simulink model "FP_PMSM_ProposedDTC"  (R2023b)
settings: Solver=ode1  StartTime=0.0  StopTime=2  FixedStep=140e-6  RelTol=1e-3
undefined symbols (not defined in the file): J, Lamda_PM, Lls, Ls, Mod_Lamda_s_ref, P, Rs
libraries: spsPWMGeneratorDCDCLib x1, spspowerguiLib x1
(part 1 of 2)
settings Model: SimulationMode=rapid-accelerator  Creator=rajan  LastModifiedBy=rajan
settings SolverCC: AlgebraicLoopSolver=TrustRegion
settings DataIOCC: ReturnWorkspaceOutputs=off
settings OptimizationCC: BlockReduction=off
settings DebuggingCC: AlgebraicLoopMsg=none  UnconnectedInputMsg=warning  UnconnectedOutputMsg=warning  UnconnectedLineMsg=warning  ArithmeticOperatorsInVariantConditions=warning
settings ModelReferenceCC: EnableRefExpFcnMdlSchedulingChecks=on
settings SFSimCC: SimUseLocalCustomCode=off  CustomCodeUndefinedFunction=UseInterfaceOnly
settings RTWCC: RTWUseLocalCustomCode=off
settings CodeAppCC: StateflowObjectComments=on
settings SimscapeCC: SimscapeNormalizeSystem=off

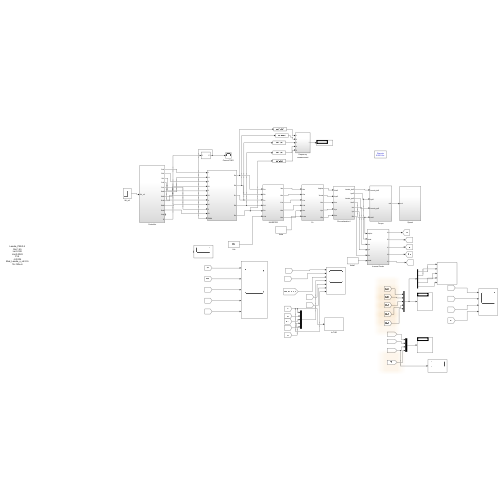
[thumbnail: Simulink's stored preview of the top-level diagram]
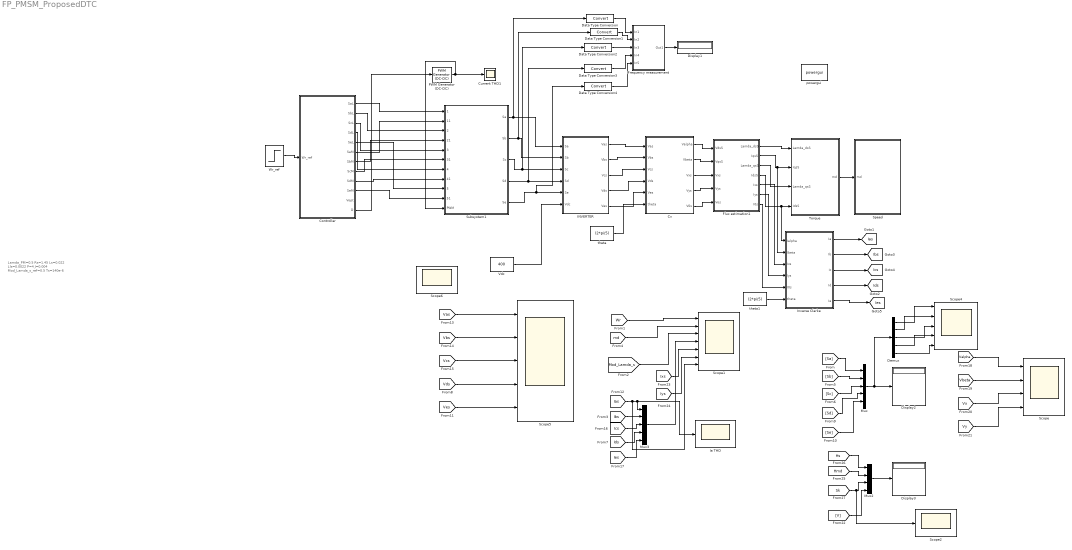
== system FP_PMSM_ProposedDTC ==
  note: Lamda_PM=0.5
      | Rs=1.45
      | Ls=0.022
      | Lls=0.0022
      | P=4
      | J=0.004
      | Mod_Lamda_s_ref=0.5
      | Ts=140e-6
  Controller : Subsystem
  Current THD1 : Scope
  "Cv " : Subsystem
  Data Type Conversion{,1..4} (5 alike) : DataTypeConversion  SaturateOnIntegerOverflow=off  RndMeth=Floor
  Demux : Demux  Outputs=5
  Display1 : Display
  Display2 : Display
  Display3 : Display
  Flux estimation1 : Subsystem
  Frequency measurement : Subsystem
  INVERTER : Subsystem
  Ia THD : Scope
  Inverse Clarke : Subsystem
  Mux : Mux  Inputs=5
  Mux2 : Mux
  Mux3 : Mux  Inputs=5
  PWM Generator (DC-DC) : spsPWMGeneratorDCDCLib/PWM Generator (DC-DC)  Fsw=3000  Ts=140e-6
  Scope : Scope  NumInputPorts=4
  Scope1 : Scope  NumInputPorts=7
  Scope2 : Scope
  Scope4 : Scope  NumInputPorts=5
  Scope5 : Scope  NumInputPorts=5
  Scope6 : Scope
  Speed : Subsystem
  Subsystem1 : Subsystem
  Torque : Subsystem
  Vdc : Constant  Value=400
  Wr_ref : Step  Time=0.5  Before=104.7197  After=104.7197  SampleTime=0  VectorParams1D=off
  powergui : spspowerguiLib/powergui  Priority=1  SimulationMode=Discrete  SampleTime=140e-6  frequency=60  Iterations=50  frequencyindice=60  Pbase=100e6  ErrMax=1e-4  UnitsV=kV  UnitsW=MW  buscounter=0  FunctionMessages=off  echomessages=off  EnableUseOfTLC=off  CurrentSourceSwitches=off  DisableSnubberDevices=off  DisableRonSwitches=off  DisableVfSwitches=off  DisplayEquations=off  AutomaticDiscreteSolvers=off  SolverType=Tustin/Backward Euler (TBE)  Interpol=off  ExternalGateDelay=off  methode=off  Ts=10  x0status=blocks  SPID=off  SwTol=0  HookPort=off  NonlinearTolerance=1e-4  nMaxIteration=100  ContinueOnMaxIteration=off  RestoreLinks=warning  ResistiveCurrentMeasurement=off  Frange=[0:2:500]  Ylog=off  Xlog=on  ShowGrid=off  save=off  variable=ZData  structure=Ia_THD  ZoomFFT=off  StartTime=0.15  cycles=10  DisplayStyle=2  fundamental=31.83  FreqAxis=off  MaxFrequency=1000  frequencyindicesteady=1  RmsSteady=1  display=off
  theta : Constant  Value=(2*pi/5)
  theta1 : Constant  Value=(2*pi/5)
  tag scope: Ias=global, Ibs=global, Ics=global, Ids=global, Ies=global
  wires:
  [Vbs] -> Scope5/2
  [Vas] -> Scope5/1
  [Vcs] -> Scope5/3
  [Wr] -> Scope1/1
  [md] -> Scope1/2
  [Mod_Lamda_s] -> Scope1/3
  Mux2/1 -> Display3/1
  [V] -> Mux2/4
  [Hmd] -> Mux2/2
  [Hs] -> Mux2/1
  [Sk] -> Scope2/1, Mux2/3
  [Ics] -> Mux3/3
  [Ias] -> Scope1/7, Mux3/1, Ia THD/1
  [Ibs] -> Mux3/2
  [Ids] -> Mux3/4
  [Ies] -> Mux3/5
  Mux3/1 -> Scope1/4
  INVERTER/1(Vas) -> "Cv "/1(Vas)
  INVERTER/2(Vbs) -> "Cv "/2(Vbs)
  INVERTER/3(Vcs) -> "Cv "/3(Vcs)
  INVERTER/4(Vds) -> "Cv "/4(Vds)
  INVERTER/5(Ves) -> "Cv "/5(Ves)
  "Cv "/1(Valpha) -> Flux estimation1/1(VdsS)
  "Cv "/2(Vbeta) -> Flux estimation1/2(VqsS)
  Flux estimation1/1(Lamda_dsS) -> Torque/1(Lamda_dsS)
  Flux estimation1/2(IqsS) -> Torque/2(IqsS), Inverse Clarke/2(Ibeta)
  Flux estimation1/3(Lamda_qsS) -> Torque/3(Lamda_qsS)
  Flux estimation1/4(IdsS) -> Inverse Clarke/1(Ialpha), Torque/4(IdsS)
  Torque/1(md) -> Speed/1(md)
  Wr_ref/1 -> Controller/1(Wr_ref)
  [Vds] -> Scope5/4
  [Ves] -> Scope5/5
  Vdc/1 -> INVERTER/6(Vdc)
  theta/1 -> "Cv "/6(theta)
  "Cv "/3(Vxs) -> Flux estimation1/3(Vxs)
  "Cv "/4(Vys) -> Flux estimation1/4(Vys)
  "Cv "/5(V0s) -> Flux estimation1/5(Vos)
  [Valpha] -> Scope/1
  [Vbeta] -> Scope/2
  [Vx] -> Scope/3
  [Vy] -> Scope/4
  [Ixs] -> Scope1/5
  [Iys] -> Scope1/6
  Flux estimation1/5(Ixs) -> Inverse Clarke/3(Ixs)
  Flux estimation1/6(Iys) -> Inverse Clarke/4(Iys)
  Flux estimation1/7(I0s) -> Inverse Clarke/5(I0s)
  theta1/1 -> Inverse Clarke/6(theta)
  Inverse Clarke/1(Ia) -> [Ias]
  Inverse Clarke/2(Ib) -> [Ibs]
  Inverse Clarke/3(Ic) -> [Ics]
  Inverse Clarke/4(Id) -> [Ids]
  Inverse Clarke/5(Ie) -> [Ies]
  [Sa] -> Mux/1
  [Sb] -> Mux/2
  [Sc] -> Mux/3
  Mux/1 -> Demux/1, Display2/1
  [Sd] -> Mux/4
  [Se] -> Mux/5
  Demux/1 -> Scope4/1
  Demux/2 -> Scope4/2
  Demux/3 -> Scope4/3
  Demux/4 -> Scope4/4
  Demux/5 -> Scope4/5
  PWM Generator (DC-DC)/1 -> Subsystem1/11(PWM), Current THD1/1
  Controller/1(SaL) -> Subsystem1/1(1)
  Controller/2(SbL) -> Subsystem1/3(2)
  Controller/3(ScL) -> Subsystem1/5(3)
  Controller/4(SdL) -> Subsystem1/7(4)
  Controller/5(SeL) -> Subsystem1/9(5)
  Controller/6(SaM) -> Subsystem1/2(11)
  Controller/7(SbM) -> Subsystem1/4(21)
  Controller/8(ScM) -> Subsystem1/6(31)
  Controller/9(SdM) -> Subsystem1/8(41)
  Controller/10(SeM) -> Subsystem1/10(51)
  Controller/12(D) -> PWM Generator (DC-DC)/1
  Subsystem1/1(Sa) -> Data Type Conversion/1, INVERTER/1(Sa)
  Subsystem1/2(Sb) -> Data Type Conversion1/1, INVERTER/2(Sb)
  Subsystem1/3(Sc) -> Data Type Conversion2/1, INVERTER/3(Sc)
  Subsystem1/4(Sd) -> Data Type Conversion3/1, INVERTER/4(Sd)
  Subsystem1/5(Se) -> Data Type Conversion4/1, INVERTER/5(Se)
  Frequency measurement/1(Out1) -> Display1/1
  Data Type Conversion/1 -> Frequency measurement/1(In1)
  Data Type Conversion1/1 -> Frequency measurement/2(In2)
  Data Type Conversion2/1 -> Frequency measurement/3(In3)
  Data Type Conversion3/1 -> Frequency measurement/4(In4)
  Data Type Conversion4/1 -> Frequency measurement/5(In5)

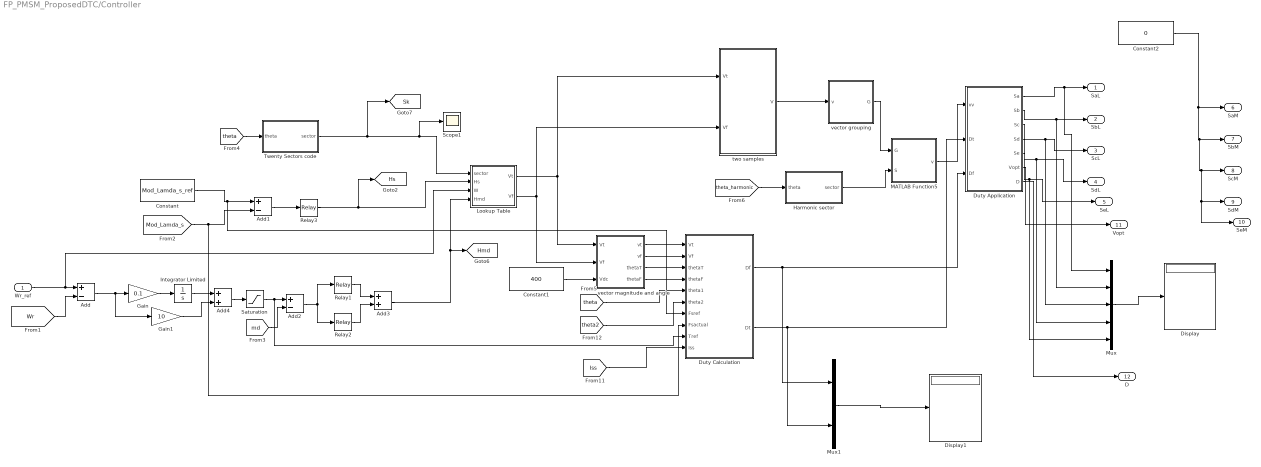
== system FP_PMSM_ProposedDTC/Controller ==
  Wr_ref : Inport
  Add : Sum  Inputs=+-
  Add1 : Sum  Inputs=+-
  Add2 : Sum  Inputs=+-
  Add3 : Sum
  Add4 : Sum
  Constant : Constant  Value=Mod_Lamda_s_ref
  Constant1 : Constant  Value=400
  Constant2 : Constant  Value=0
  Display : Display
  Display1 : Display
  Duty Application : MATLAB Function  TreatAsAtomicUnit=on
  Duty Calculation : MATLAB Function  TreatAsAtomicUnit=on
  Gain : Gain  Gain=0.1
  Gain1 : Gain  Gain=10
  "Harmonic sector " : MATLAB Function  TreatAsAtomicUnit=on
  Integrator Limited : Integrator  LimitOutput=on  UpperSaturationLimit=14  LowerSaturationLimit=-14
  Lookup Table : MATLAB Function  TreatAsAtomicUnit=on
  MATLAB Function5 : MATLAB Function  TreatAsAtomicUnit=on
  Mux : Mux  Inputs=5
  Mux1 : Mux  Inputs=2
  Relay1 : Relay  OnSwitchValue=1.4  OffSwitchValue=0
  Relay2 : Relay  OnSwitchValue=0  OffSwitchValue=-1.4  OnOutputValue=0  OffOutputValue=-1
  Relay3 : Relay  OnSwitchValue=0.005  OffSwitchValue=-0.005  OffOutputValue=-1
  Saturation : Saturate  UpperLimit=14  LowerLimit=-14
  Scope1 : Scope
  Twenty Sectors code : MATLAB Function  TreatAsAtomicUnit=on
  two samples : MATLAB Function  TreatAsAtomicUnit=on
  vector grouping : MATLAB Function  TreatAsAtomicUnit=on
  vector magnitude and angle : Subsystem
  SaL : Outport
  SbL : Outport  Port=2
  ScL : Outport  Port=3
  SdL : Outport  Port=4
  SeL : Outport  Port=5
  SaM : Outport  Port=6
  SbM : Outport  Port=7
  ScM : Outport  Port=8
  SdM : Outport  Port=9
  SeM : Outport  Port=10
  Vopt : Outport  Port=11
  D : Outport  Port=12
  tag scope: Hmd=global, Hs=global, Sk=global
  wires:
  Gain1/1 -> Add4/2
  Integrator Limited/1 -> Add4/1
  [md] -> Add2/2
  Gain/1 -> Integrator Limited/1
  Relay2/1 -> Add3/2
  [Wr] -> Add/2
  Add1/1 -> Relay3/1
  Relay3/1 -> Lookup Table/2(Hs), [Hs]
  [theta] -> Twenty Sectors code/1(theta)
  Constant/1 -> Duty Calculation/7(Fsref), Add1/1
  Add3/1 -> Lookup Table/4(Hmd), [Hmd]
  [Mod_Lamda_s] -> Duty Calculation/8(Fsactual), Add1/2
  Add2/1 -> Relay1/1, Relay2/1
  Relay1/1 -> Add3/1
  Add/1 -> Gain1/1, Gain/1
  Saturation/1 -> Duty Calculation/9(Tref), Add2/1
  Add4/1 -> Saturation/1
  Wr_ref/1 -> Lookup Table/3(W), Add/1
  Twenty Sectors code/1(sector) -> [Sk], Lookup Table/1(sector), Scope1/1
  Lookup Table/1(Vt) -> vector magnitude and angle/1(Vt), two samples/1(Vt)
  Lookup Table/2(Vf) -> vector magnitude and angle/2(Vf), two samples/2(Vf)
  Constant1/1 -> vector magnitude and angle/3(Vdc)
  vector magnitude and angle/1(vt) -> Duty Calculation/1(Vt)
  vector magnitude and angle/2(vf) -> Duty Calculation/2(Vf)
  vector magnitude and angle/3(thetaT) -> Duty Calculation/3(thetaT)
  vector magnitude and angle/4(thetaF) -> Duty Calculation/4(thetaF)
  [theta] -> Duty Calculation/5(theta1)
  [theta2] -> Duty Calculation/6(theta2)
  [Iss] -> Duty Calculation/10(Iss)
  "Harmonic sector "/1(sector) -> MATLAB Function5/2(S)
  vector grouping/1(G) -> MATLAB Function5/1(G)
  MATLAB Function5/1(v) -> Duty Application/1(vv)
  [theta_harmonic] -> "Harmonic sector "/1(theta)
  two samples/1(V) -> vector grouping/1(v)
  Duty Application/1(Sa) -> Mux/1, SaL/1
  Duty Application/2(Sb) -> Mux/2, SbL/1
  Duty Application/3(Sc) -> Mux/3, ScL/1
  Duty Application/4(Sd) -> Mux/4, SdL/1
  Duty Application/5(Se) -> Mux/5, SeL/1
  Duty Calculation/2(Dt) -> Mux1/2, Duty Application/2(Dt)
  Duty Calculation/1(Df) -> Mux1/1, Duty Application/3(Df)
  Mux/1 -> Display/1
  Mux1/1 -> Display1/1
  Duty Application/6(Vopt) -> Vopt/1
  Constant2/1 -> SeM/1, SdM/1, ScM/1, SbM/1, SaM/1
  Duty Application/7(D) -> D/1

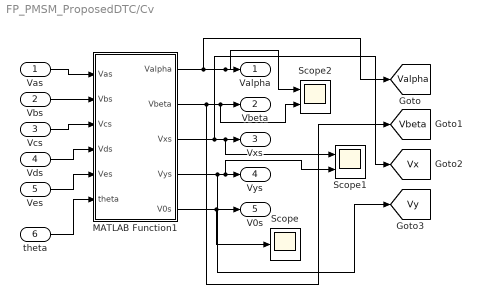
== system FP_PMSM_ProposedDTC/Cv  ==
  Vas : Inport
  Vbs : Inport  Port=2
  Vcs : Inport  Port=3
  Vds : Inport  Port=4
  Ves : Inport  Port=5
  theta : Inport  Port=6
  MATLAB Function1 : MATLAB Function  TreatAsAtomicUnit=on
  Scope : Scope
  Scope1 : Scope  NumInputPorts=2
  Scope2 : Scope  NumInputPorts=2
  Valpha : Outport
  Vbeta : Outport  Port=2
  Vxs : Outport  Port=3
  Vys : Outport  Port=4
  V0s : Outport  Port=5
  tag scope: Valpha=global, Vbeta=global, Vx=global, Vy=global
  wires:
  Vas/1 -> MATLAB Function1/1(Vas)
  Vbs/1 -> MATLAB Function1/2(Vbs)
  Ves/1 -> MATLAB Function1/5(Ves)
  Vcs/1 -> MATLAB Function1/3(Vcs)
  Vds/1 -> MATLAB Function1/4(Vds)
  theta/1 -> MATLAB Function1/6(theta)
  MATLAB Function1/1(Valpha) -> [Valpha], Scope2/1, Valpha/1
  MATLAB Function1/2(Vbeta) -> [Vbeta], Scope2/2, Vbeta/1
  MATLAB Function1/3(Vxs) -> [Vx], Scope1/1, Vxs/1
  MATLAB Function1/4(Vys) -> Vys/1, Scope1/2, [Vy]
  MATLAB Function1/5(V0s) -> Scope/1, V0s/1

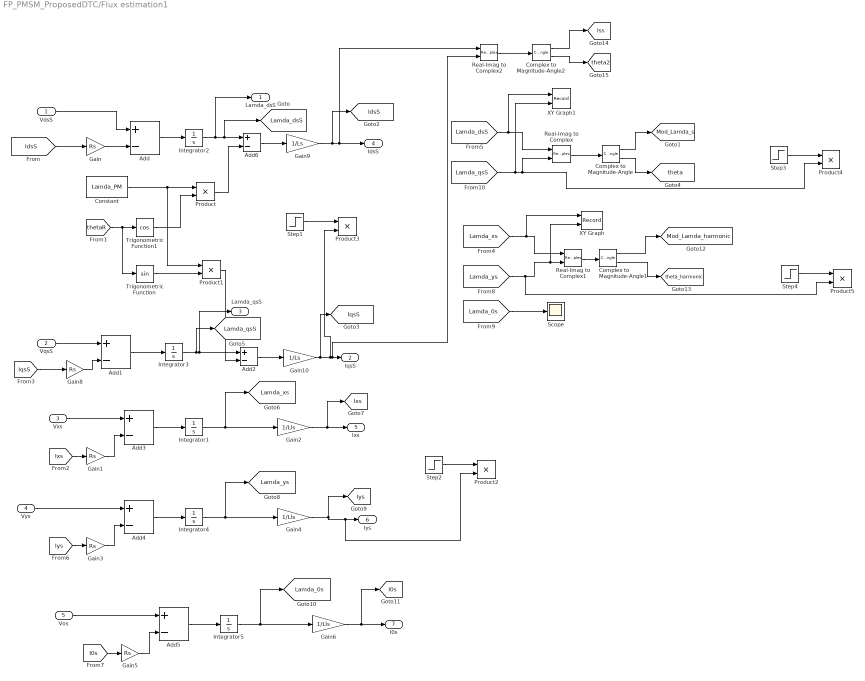
== system FP_PMSM_ProposedDTC/Flux estimation1 ==
  VdsS : Inport
  VqsS : Inport  Port=2
  Vxs : Inport  Port=3
  Vys : Inport  Port=4
  Vos : Inport  Port=5
  Add{,1..6} (7 alike) : Sum  Inputs=+-
  Complex to Magnitude-Angle : ComplexToMagnitudeAngle
  Complex to Magnitude-Angle1 : ComplexToMagnitudeAngle
  Complex to Magnitude-Angle2 : ComplexToMagnitudeAngle
  Constant : Constant  Value=Lamda_PM
  Gain{,1,3,5,8} (5 alike) : Gain  Gain=Rs
  Gain10 : Gain  Gain=1/Ls
  Gain2 : Gain  Gain=1/Lls
  Gain4 : Gain  Gain=1/Lls
  Gain6 : Gain  Gain=1/Lls
  Gain9 : Gain  Gain=1/Ls
  Integrator{1..5} (5 alike) : Integrator  UpperSaturationLimit=0.5  LowerSaturationLimit=-0.5
  Product{,1..5} (6 alike) : Product
  Real-Imag to Complex : RealImagToComplex
  Real-Imag to Complex1 : RealImagToComplex
  Real-Imag to Complex2 : RealImagToComplex
  Scope : Scope
  Step{1..4} (4 alike) : Step  Time=0.5  SampleTime=0
  Trigonometric Function : Trigonometry
  Trigonometric Function1 : Trigonometry  Operator=cos
  XY Graph : Record  FileSettingsInternal="{\"entries\":[{\"content\":{\"excelSettings\":{\"content\":{},\"type\":\"Streamout.ExcelSettings\"}},\"type\":\"Streamout.FileSettingStorage\",\"uuid\":\"\"}],\"packageUris\":[\"http:\\/\\/schema.mathworks.com\\/mf0\\/streamout_blocks\\/R2020a\"],\"version\":\"1.0\"}"  Layout=[1 1]  SignalsInternal="{\"entries\":[{\"content\":{\"signals\":[{\"content\":{\"blockPath\":[],\"dimensions\":[1],\"domain\":\"\",\"lineColor\":\"#a2142f\",\"plots\":[1],\"port\":1,\"signalID\":24,\"signalName\":\"XY Graph:1\"},\"type\":\"RecordBlkView.Signal\",\"uuid\":\"\"},{\"content\":{\"blockPath\":[],\"dimensions\":[1],\"domain\":\"\",\"lineColor\":\"#139fff\",\"plots\":[1],\"port\":2,\"signalID\":27,\"signalName\":\"XY Graph:2\"},\"type\":\"RecordBlkView.Signal\",\"uuid\":\"\"}]},\"type\":\"RecordBlkView.InputSignals\",\"uuid\":\"\"}],\"packageUris\":[\"http:\\/\\/schema.mathworks.com\\/mf0\\/streamout_blocks\\/R2020a\"],\"version\":\"1.0\"}"  VisualizationBindings="{\"xyplotplugin\":{\"info\":[{\"series\":[{\"bindingParametersList\":[{\"parameter\":\"X-Axis\",\"signalID\":24,\"signalName\":\"XY Graph:1\"},{\"parameter\":\"Y-Axis\",\"signalID\":27,\"signalName\":\"XY Graph:2\"}],\"seriesID\":36795}],\"subplotID\":1}]}}"  CompatibilityTag=XY  st=-1
  XY Graph1 : Record  FileSettingsInternal="{\"entries\":[{\"content\":{\"excelSettings\":{\"content\":{},\"type\":\"Streamout.ExcelSettings\"}},\"type\":\"Streamout.FileSettingStorage\",\"uuid\":\"\"}],\"packageUris\":[\"http:\\/\\/schema.mathworks.com\\/mf0\\/streamout_blocks\\/R2020a\"],\"version\":\"1.0\"}"  Layout=[1 1]  SignalsInternal="{\"entries\":[{\"content\":{\"signals\":[{\"content\":{\"blockPath\":[],\"dimensions\":[1],\"domain\":\"\",\"lineColor\":\"#a2142f\",\"plots\":[1],\"port\":1,\"signalID\":16,\"signalName\":\"XY Graph:1\"},\"type\":\"RecordBlkView.Signal\",\"uuid\":\"\"},{\"content\":{\"blockPath\":[],\"dimensions\":[1],\"domain\":\"\",\"lineColor\":\"#139fff\",\"plots\":[1],\"port\":2,\"signalID\":19,\"signalName\":\"XY Graph:2\"},\"type\":\"RecordBlkView.Signal\",\"uuid\":\"\"}]},\"type\":\"RecordBlkView.InputSignals\",\"uuid\":\"\"}],\"packageUris\":[\"http:\\/\\/schema.mathworks.com\\/mf0\\/streamout_blocks\\/R2020a\"],\"version\":\"1.0\"}"  VisualizationBindings="{\"xyplotplugin\":{\"info\":[{\"series\":[{\"bindingParametersList\":[{\"parameter\":\"X-Axis\",\"signalID\":16,\"signalName\":\"XY Graph:1\"},{\"parameter\":\"Y-Axis\",\"signalID\":19,\"signalName\":\"XY Graph:2\"}],\"seriesID\":10148}],\"subplotID\":1}]}}"  CompatibilityTag=XY  st=-1
  Lamda_dsS : Outport
  IqsS : Outport  Port=2
  Lamda_qsS : Outport  Port=3
  IdsS : Outport  Port=4
  Ixs : Outport  Port=5
  Iys : Outport  Port=6
  I0s : Outport  Port=7
  tag scope: I0s=global, IdsS=global, IqsS=global, Iss=global, Ixs=global, Iys=global, Lamda_0s=global, Lamda_dsS=global, Lamda_qsS=global, Lamda_xs=global, Lamda_ys=global, Mod_Lamda_harmonic=global, Mod_Lamda_s=global, theta2=global, theta=global, theta_harmonic=global
  wires:
  Real-Imag to Complex/1 -> Complex to Magnitude-Angle/1
  Complex to Magnitude-Angle/1 -> [Mod_Lamda_s]
  Add/1 -> Integrator2/1
  Integrator2/1 -> Lamda_dsS/1, [Lamda_dsS], Add6/1
  VqsS/1 -> Add1/1
  Add1/1 -> Integrator3/1
  Integrator3/1 -> [Lamda_qsS], Add2/1, Lamda_qsS/1
  Gain8/1 -> Add1/2
  [IdsS] -> Gain/1
  Gain/1 -> Add/2
  VdsS/1 -> Add/1
  [IqsS] -> Gain8/1
  Add6/1 -> Gain9/1
  Complex to Magnitude-Angle/2 -> [theta]
  Add2/1 -> Gain10/1
  [thetaR] -> Trigonometric Function/1, Trigonometric Function1/1
  Constant/1 -> Product1/1, Product/1
  Trigonometric Function1/1 -> Product/2
  Product/1 -> Add6/2
  Trigonometric Function/1 -> Product1/2
  Product1/1 -> Add2/2
  [Ixs] -> Gain1/1
  Gain1/1 -> Add3/2
  Vxs/1 -> Add3/1
  Add3/1 -> Integrator1/1
  Integrator1/1 -> [Lamda_xs], Gain2/1
  Add4/1 -> Integrator4/1
  Vys/1 -> Add4/1
  [Iys] -> Gain3/1
  Gain3/1 -> Add4/2
  Integrator4/1 -> [Lamda_ys], Gain4/1
  Gain5/1 -> Add5/2
  Gain6/1 -> I0s/1, [I0s]
  Vos/1 -> Add5/1
  Integrator5/1 -> [Lamda_0s], Gain6/1
  Add5/1 -> Integrator5/1
  [I0s] -> Gain5/1
  Complex to Magnitude-Angle1/1 -> [Mod_Lamda_harmonic]
  Complex to Magnitude-Angle1/2 -> [theta_harmonic]
  Real-Imag to Complex1/1 -> Complex to Magnitude-Angle1/1
  [Lamda_0s] -> Scope/1
  Step1/1 -> Product3/1
  Gain4/1 -> [Iys], Product2/2, Iys/1
  Step2/1 -> Product2/1
  Gain2/1 -> Ixs/1, [Ixs]
  [Lamda_qsS] -> XY Graph1/2, Product4/2, Real-Imag to Complex/2
  Step3/1 -> Product4/1
  [Lamda_dsS] -> XY Graph1/1, Real-Imag to Complex/1
  [Lamda_ys] -> Product5/2, XY Graph/2, Real-Imag to Complex1/2
  Step4/1 -> Product5/1
  [Lamda_xs] -> Real-Imag to Complex1/1, XY Graph/1
  Gain9/1 -> [IdsS], Real-Imag to Complex2/1, IdsS/1
  Gain10/1 -> [IqsS], Product3/2, Real-Imag to Complex2/2, IqsS/1
  Real-Imag to Complex2/1 -> Complex to Magnitude-Angle2/1
  Complex to Magnitude-Angle2/1 -> [Iss]
  Complex to Magnitude-Angle2/2 -> [theta2]

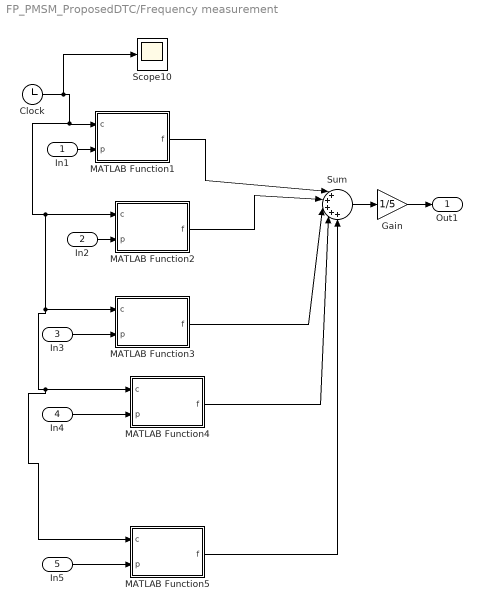
== system FP_PMSM_ProposedDTC/Frequency measurement ==
  In1 : Inport
  In2 : Inport  Port=2
  In3 : Inport  Port=3
  In4 : Inport  Port=4
  In5 : Inport  Port=5
  Clock : Clock
  Gain : Gain  Gain=1/5
  MATLAB Function1 : MATLAB Function  TreatAsAtomicUnit=on
  MATLAB Function2 : MATLAB Function  TreatAsAtomicUnit=on
  MATLAB Function3 : MATLAB Function  TreatAsAtomicUnit=on
  MATLAB Function4 : MATLAB Function  TreatAsAtomicUnit=on
  MATLAB Function5 : MATLAB Function  TreatAsAtomicUnit=on
  Scope10 : Scope
  Sum : Sum  Inputs=|+++++
  Out1 : Outport
  wires:
  MATLAB Function1/1(f) -> Sum/1
  In1/1 -> MATLAB Function1/2(p)
  MATLAB Function2/1(f) -> Sum/2
  In2/1 -> MATLAB Function2/2(p)
  MATLAB Function3/1(f) -> Sum/3
  In3/1 -> MATLAB Function3/2(p)
  Sum/1 -> Gain/1
  Gain/1 -> Out1/1
  MATLAB Function4/1(f) -> Sum/4
  In4/1 -> MATLAB Function4/2(p)
  Clock/1 -> Scope10/1, MATLAB Function5/1(c), MATLAB Function4/1(c), MATLAB Function3/1(c), MATLAB Function2/1(c), MATLAB Function1/1(c)
  MATLAB Function5/1(f) -> Sum/5
  In5/1 -> MATLAB Function5/2(p)

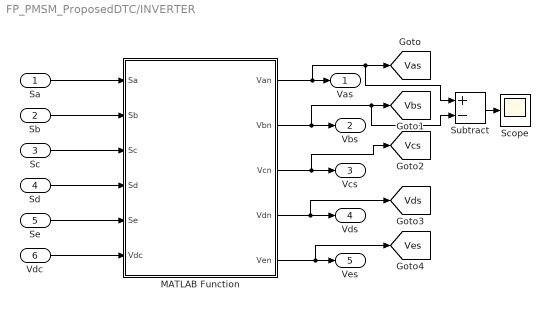
== system FP_PMSM_ProposedDTC/INVERTER ==
  Sa : Inport
  Sb : Inport  Port=2
  Sc : Inport  Port=3
  Sd : Inport  Port=4
  Se : Inport  Port=5
  Vdc : Inport  Port=6
  MATLAB Function : MATLAB Function  TreatAsAtomicUnit=on
  Scope : Scope
  Subtract : Sum  Inputs=+-
  Vas : Outport
  Vbs : Outport  Port=2
  Vcs : Outport  Port=3
  Vds : Outport  Port=4
  Ves : Outport  Port=5
  tag scope: Vas=global, Vbs=global, Vcs=global, Vds=global, Ves=global
  wires:
  MATLAB Function/1(Van) -> Subtract/1, [Vas], Vas/1
  MATLAB Function/3(Vcn) -> [Vcs], Vcs/1
  MATLAB Function/4(Vdn) -> [Vds], Vds/1
  Sc/1 -> MATLAB Function/3(Sc)
  Sa/1 -> MATLAB Function/1(Sa)
  Sb/1 -> MATLAB Function/2(Sb)
  Sd/1 -> MATLAB Function/4(Sd)
  Se/1 -> MATLAB Function/5(Se)
  Vdc/1 -> MATLAB Function/6(Vdc)
  MATLAB Function/2(Vbn) -> Subtract/2, [Vbs], Vbs/1
  MATLAB Function/5(Ven) -> [Ves], Ves/1
  Subtract/1 -> Scope/1

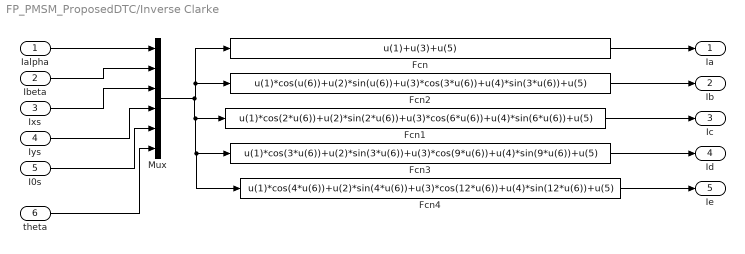
== system FP_PMSM_ProposedDTC/Inverse Clarke ==
  Ialpha : Inport
  Ibeta : Inport  Port=2
  Ixs : Inport  Port=3
  Iys : Inport  Port=4
  I0s : Inport  Port=5
  theta : Inport  Port=6
  Fcn : Fcn  Expr=u(1)+u(3)+u(5)
  Fcn1 : Fcn  Expr=u(1)*cos(2*u(6))+u(2)*sin(2*u(6))+u(3)*cos(6*u(6))+u(4)*sin(6*u(6))+u(5)
  Fcn2 : Fcn  Expr=u(1)*cos(u(6))+u(2)*sin(u(6))+u(3)*cos(3*u(6))+u(4)*sin(3*u(6))+u(5)
  Fcn3 : Fcn  Expr=u(1)*cos(3*u(6))+u(2)*sin(3*u(6))+u(3)*cos(9*u(6))+u(4)*sin(9*u(6))+u(5)
  Fcn4 : Fcn  Expr=u(1)*cos(4*u(6))+u(2)*sin(4*u(6))+u(3)*cos(12*u(6))+u(4)*sin(12*u(6))+u(5)
  Mux : Mux  Inputs=6
  Ia : Outport
  Ib : Outport  Port=2
  Ic : Outport  Port=3
  Id : Outport  Port=4
  Ie : Outport  Port=5
  wires:
  Ialpha/1 -> Mux/1
  Ibeta/1 -> Mux/2
  Ixs/1 -> Mux/3
  Iys/1 -> Mux/4
  I0s/1 -> Mux/5
  theta/1 -> Mux/6
  Fcn/1 -> Ia/1
  Mux/1 -> Fcn1/1, Fcn4/1, Fcn3/1, Fcn2/1, Fcn/1
  Fcn2/1 -> Ib/1
  Fcn1/1 -> Ic/1
  Fcn3/1 -> Id/1
  Fcn4/1 -> Ie/1

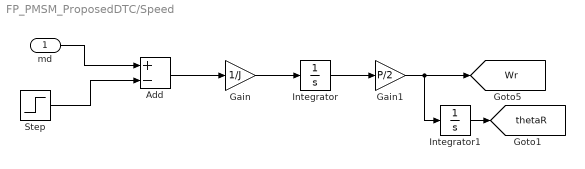
== system FP_PMSM_ProposedDTC/Speed ==
  md : Inport
  Add : Sum  Inputs=+-
  Gain : Gain  Gain=1/J
  Gain1 : Gain  Gain=P/2
  Integrator : Integrator
  Integrator1 : Integrator
  Step : Step  Time=0.1  After=0  SampleTime=0
  tag scope: Wr=global, thetaR=global
  wires:
  Gain1/1 -> Integrator1/1, [Wr]
  Add/1 -> Gain/1
  Integrator/1 -> Gain1/1
  Gain/1 -> Integrator/1
  md/1 -> Add/1
  Step/1 -> Add/2
  Integrator1/1 -> [thetaR]

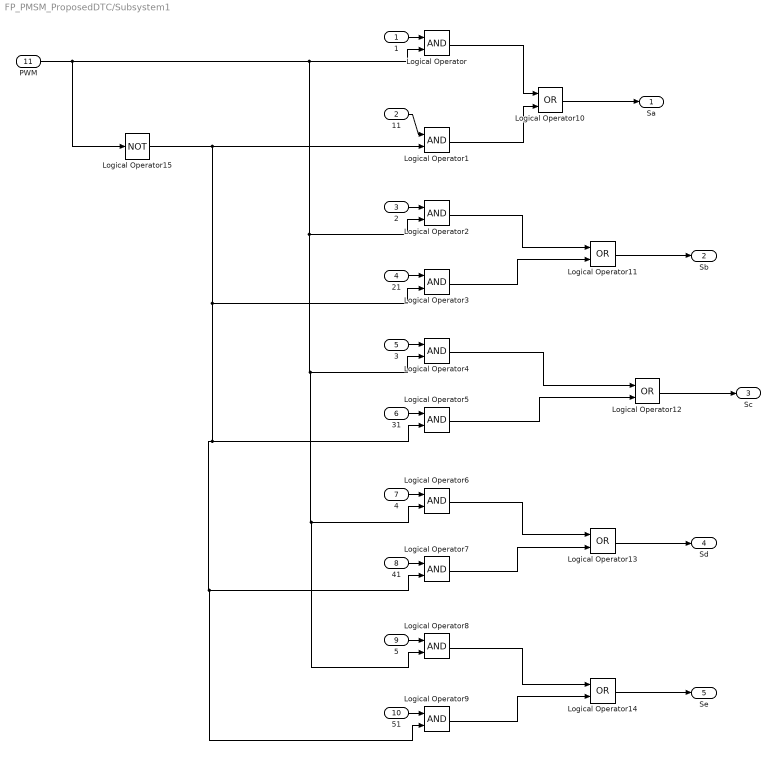
== system FP_PMSM_ProposedDTC/Subsystem1 ==
  1 : Inport
  11 : Inport  Port=2
  2 : Inport  Port=3
  21 : Inport  Port=4
  3 : Inport  Port=5
  31 : Inport  Port=6
  4 : Inport  Port=7
  41 : Inport  Port=8
  5 : Inport  Port=9
  51 : Inport  Port=10
  PWM : Inport  Port=11
  Logical Operator{,1..9} (10 alike) : Logic  AllPortsSameDT=off  OutDataTypeStr=boolean
  Logical Operator{10..14} (5 alike) : Logic  Operator=OR  AllPortsSameDT=off  OutDataTypeStr=boolean
  Logical Operator15 : Logic  Operator=NOT  AllPortsSameDT=off  OutDataTypeStr=boolean
  Sa : Outport
  Sb : Outport  Port=2
  Sc : Outport  Port=3
  Sd : Outport  Port=4
  Se : Outport  Port=5
  wires:
  PWM/1 -> Logical Operator15/1, Logical Operator2/2, Logical Operator8/2, Logical Operator6/2, Logical Operator4/2, Logical Operator/2
  1/1 -> Logical Operator/1
  5/1 -> Logical Operator8/1
  21/1 -> Logical Operator3/1
  11/1 -> Logical Operator1/1
  3/1 -> Logical Operator4/1
  2/1 -> Logical Operator2/1
  Logical Operator1/1 -> Logical Operator10/2
  4/1 -> Logical Operator6/1
  51/1 -> Logical Operator9/1
  31/1 -> Logical Operator5/1
  41/1 -> Logical Operator7/1
  Logical Operator/1 -> Logical Operator10/1
  Logical Operator10/1 -> Sa/1
  Logical Operator3/1 -> Logical Operator11/2
  Logical Operator2/1 -> Logical Operator11/1
  Logical Operator11/1 -> Sb/1
  Logical Operator5/1 -> Logical Operator12/2
  Logical Operator4/1 -> Logical Operator12/1
  Logical Operator12/1 -> Sc/1
  Logical Operator7/1 -> Logical Operator13/2
  Logical Operator6/1 -> Logical Operator13/1
  Logical Operator13/1 -> Sd/1
  Logical Operator9/1 -> Logical Operator14/2
  Logical Operator14/1 -> Se/1
  Logical Operator8/1 -> Logical Operator14/1
  Logical Operator15/1 -> Logical Operator5/2, Logical Operator9/2, Logical Operator7/2, Logical Operator3/2, Logical Operator1/2

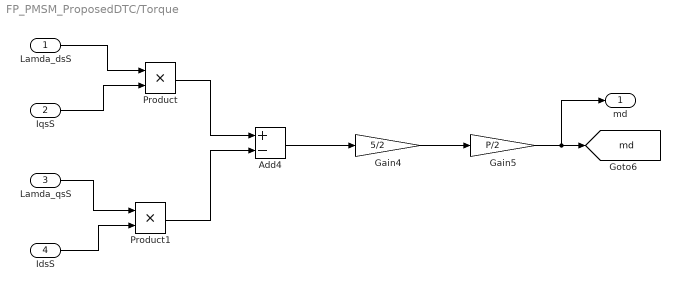
== system FP_PMSM_ProposedDTC/Torque ==
  Lamda_dsS : Inport
  IqsS : Inport  Port=2
  Lamda_qsS : Inport  Port=3
  IdsS : Inport  Port=4
  Add4 : Sum  Inputs=+-
  Gain4 : Gain  Gain=5/2
  Gain5 : Gain  Gain=P/2
  Product : Product
  Product1 : Product
  md : Outport
  tag scope: md=global
  wires:
  Lamda_dsS/1 -> Product/1
  Add4/1 -> Gain4/1
  Product/1 -> Add4/1
  Gain4/1 -> Gain5/1
  IqsS/1 -> Product/2
  IdsS/1 -> Product1/2
  Gain5/1 -> md/1, [md]
  Lamda_qsS/1 -> Product1/1
  Product1/1 -> Add4/2

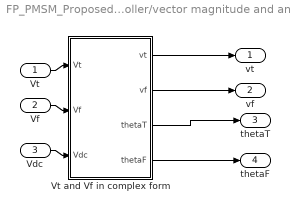
== system FP_PMSM_ProposedDTC/Controller/vector magnitude and angle ==
  Vt : Inport
  Vf : Inport  Port=2
  Vdc : Inport  Port=3
  Vt and Vf in complex form : MATLAB Function  TreatAsAtomicUnit=on
  vt : Outport
  vf : Outport  Port=2
  thetaT : Outport  Port=3
  thetaF : Outport  Port=4
  wires:
  Vf/1 -> Vt and Vf in complex form/2(Vf)
  Vt/1 -> Vt and Vf in complex form/1(Vt)
  Vdc/1 -> Vt and Vf in complex form/3(Vdc)
  Vt and Vf in complex form/1(vt) -> vt/1
  Vt and Vf in complex form/2(vf) -> vf/1
  Vt and Vf in complex form/3(thetaT) -> thetaT/1
  Vt and Vf in complex form/4(thetaF) -> thetaF/1

== matlab function FP_PMSM_ProposedDTC/Controller/vector grouping ==
  data: v input; G output
function G  = fcn(v)
% low speed of operation
if (v==1) || (v==11) ||(v==21) 
     G=1;
elseif(v==2) || (v==12) ||(v==22) 
     G=2;
elseif(v==3) || (v==13) ||(v==23) 
     G=3;
 elseif(v==4) ||(v==14) ||(v==24) 
     G=4;   
 elseif(v==5) || (v==15) ||(v==25) 
     G=5;   
elseif(v==6) || (v==16) ||(v==26) 
     G=6;
elseif(v==7) || (v==17) ||(v==27) 
     G=7;
elseif(v==8) || (v==18) ||(v==28) 
     G=8;
elseif(v==9) || (v==19) ||(v==29) 
     G=9;
else
     G=10;
end

== matlab function FP_PMSM_ProposedDTC/Cv /MATLAB Function1 ==
  data: Vas input; Valpha output; Vbs input; Vcs input; Vds input; Ves input; theta input; Vbeta output; Vxs output; Vys output; V0s output
function [Valpha,Vbeta,Vxs,Vys,V0s] = fcn(Vas,Vbs,Vcs,Vds,Ves,theta)
Valpha=(2/5)*(Vas*cos(0)+Vbs*cos(theta)+Vcs*cos(2*theta)+Vds*cos(3*theta)+Ves*cos(4*theta));
Vbeta=(2/5)*(Vas*sin(0)+Vbs*sin(theta)+Vcs*sin(2*theta)+Vds*sin(3*theta)+Ves*sin(4*theta));
Vxs=(2/5)*(Vas*cos(0)+Vbs*cos(3*theta)+Vcs*cos(6*theta)+Vds*cos(9*theta)+Ves*cos(12*theta));
Vys=(2/5)*(Vas*sin(0)+Vbs*sin(3*theta)+Vcs*sin(6*theta)+Vds*sin(9*theta)+Ves*sin(12*theta));
V0s=(2/5)*(1/2)*(Vas+Vbs+Vcs+Vds+Ves);

== matlab function FP_PMSM_ProposedDTC/Controller/Lookup Table ==
  data: sector input; Vt output; Hs input; W input; Hmd input; Vf output
function [Vt,Vf]=fcn(sector,Hs,W,Hmd)
%#codegen
Vt=0;
Vf=0;
% low speed of operation
if(abs(W)>0 && abs(W)<=100)
 if(sector==1)
     if(Hs==1 && Hmd==1)
        Vt=24;
        Vf=21;
     elseif(Hs==1 && Hmd==0)
        Vt=31;
        Vf=31;
    elseif(Hs==1 && Hmd==-1)
        Vt=29;
        Vf=21;
    elseif(Hs==-1 && Hmd==1)
        Vt=24;
        Vf=26;
    elseif(Hs==-1 && Hmd==0)
        Vt=0;
        Vf=0;
    else
        Vt=29;
        Vf=26;
    end
 end
if(sector==2)
    if(Hs==1 && Hmd==1)
        Vt=24;
        Vf=22;
     elseif(Hs==1 && Hmd==0)
        Vt=0;
        Vf=0;
    elseif(Hs==1 && Hmd==-1)
        Vt=29;
        Vf=22;
    elseif(Hs==-1 && Hmd==1)
        Vt=24;
        Vf=27;
    elseif(Hs==-1 && Hmd==0)
        Vt=31;
        Vf=31;
    else
        Vt=29;
        Vf=27;
    end
end
if(sector==3)
    if(Hs==1 && Hmd==1)
        Vt=25;
        Vf=22;
     elseif(Hs==1 && Hmd==0)
        Vt=31;
        Vf=31;
    elseif(Hs==1 && Hmd==-1)
        Vt=30;
        Vf=22;
    elseif(Hs==-1 && Hmd==1)
        Vt=25;
        Vf=27;
    elseif(Hs==-1 && Hmd==0)
        Vt=0;
        Vf=0;
    else
        Vt=30;
        Vf=27;
    end
end
if(sector==4)
    if(Hs==1 && Hmd==1)
        Vt=25;
        Vf=23;
     elseif(Hs==1 && Hmd==0)
        Vt=0;
        Vf=0;
    elseif(Hs==1 && Hmd==-1)
        Vt=30;
        Vf=23;
    elseif(Hs==-1 && Hmd==1)
        Vt=25;
        Vf=28;
    elseif(Hs==-1 && Hmd==0)
        Vt=31;
        Vf=31;
    else
        Vt=30;
        Vf=28;
    end
end
if(sector==5)
    if(Hs==1 && Hmd==1)
        Vt=26;
        Vf=23;
     elseif(Hs==1 && Hmd==0)
        Vt=31;
        Vf=31;
    elseif(Hs==1 && Hmd==-1)
        Vt=21;
        Vf=23;
    elseif(Hs==-1 && Hmd==1)
        Vt=26;
        Vf=28;
    elseif(Hs==-1 && Hmd==0)
        Vt=0;
        Vf=0;
    else
        Vt=21;
        Vf=28;
    end
end
if(sector==6)
    if(Hs==1 && Hmd==1)
        Vt=26;
        Vf=24;
     elseif(Hs==1 && Hmd==0)
        Vt=0;
        Vf=0;
    elseif(Hs==1 && Hmd==-1)
        Vt=21;
        Vf=24;
    elseif(Hs==-1 && Hmd==1)
        Vt=26;
        Vf=29;
    elseif(Hs==-1 && Hmd==0)
        Vt=31;
        Vf=31;
    else
        Vt=21;
        Vf=29;
    end
end
if(sector==7)
    if(Hs==1 && Hmd==1)
        Vt=27;
        Vf=24;
     elseif(Hs==1 && Hmd==0)
        Vt=31;
        Vf=31;
    elseif(Hs==1 && Hmd==-1)
        Vt=22;
        Vf=24;
    elseif(Hs==-1 && Hmd==1)
        Vt=27;
        Vf=29;
    elseif(Hs==-1 && Hmd==0)
        Vt=0;
        Vf=0;
    else
        Vt=22;
        Vf=29;
    end
end
if(sector==8)
    if(Hs==1 && Hmd==1)
        Vt=27;
        Vf=25;
     elseif(Hs==1 && Hmd==0)
        Vt=0;
        Vf=0;
    elseif(Hs==1 && Hmd==-1)
        Vt=22;
        Vf=25;
    elseif(Hs==-1 && Hmd==1)
        Vt=27;
        Vf=30;
    elseif(Hs==-1 && Hmd==0)
        Vt=31;
        Vf=31;
    else
        Vt=22;
        Vf=30;
    end
end
if(sector==9)
    if(Hs==1 && Hmd==1)
        Vt=28;
        Vf=25;
     elseif(Hs==1 && Hmd==0)
        Vt=31;
        Vf=31;
    elseif(Hs==1 && Hmd==-1)
        Vt=23;
        Vf=25;
    elseif(Hs==-1 && Hmd==1)
        Vt=28;
        Vf=30;
    elseif(Hs==-1 && Hmd==0)
        Vt=0;
        Vf=0;
    else
        Vt=23;
        Vf=30;
    end
end
if(sector==10)
    if(Hs==1 && Hmd==1)
        Vt=28;
        Vf=26;
     elseif(Hs==1 && Hmd==0)
        Vt=0;
        Vf=0;
    elseif(Hs==1 && Hmd==-1)
        Vt=23;
        Vf=26;
    elseif(Hs==-1 && Hmd==1)
        Vt=28;
        Vf=21;
    elseif(Hs==-1 && Hmd==0)
       Vt=31;
        Vf=31;
    else
        Vt=23;
        Vf=21;
    end
end
if(sector==11)
    if(Hs==1 && Hmd==1)
        Vt=29;
        Vf=26;
     elseif(Hs==1 && Hmd==0)
        Vt=31;
        Vf=31;
    elseif(Hs==1 && Hmd==-1)
        Vt=24;
        Vf=26;
    elseif(Hs==-1 && Hmd==1)
        Vt=29;
        Vf=21;
    elseif(Hs==-1 && Hmd==0)
       Vt=0;
        Vf=0;
    else
        Vt=24;
        Vf=21;
    end
end
if(sector==12)
    if(Hs==1 && Hmd==1)
        Vt=29;
        Vf=27;
     elseif(Hs==1 && Hmd==0)
        Vt=0;
        Vf=0;
    elseif(Hs==1 && Hmd==-1)
        Vt=24;
        Vf=27;
    elseif(Hs==-1 && Hmd==1)
        Vt=29;
        Vf=22;
    elseif(Hs==-1 && Hmd==0)
       Vt=31;
        Vf=31;
    else
        Vt=24;
        Vf=22;
    end
end
if(sector==13)
    if(Hs==1 && Hmd==1)
        Vt=30;
        Vf=27;
     elseif(Hs==1 && Hmd==0)
        Vt=31;
        Vf=31;
    elseif(Hs==1 && Hmd==-1)
        Vt=25;
        Vf=27;
    elseif(Hs==-1 && Hmd==1)
        Vt=30;
        Vf=22;
    elseif(Hs==-1 && Hmd==0)
       Vt=0;
        Vf=0;
    else
        Vt=25;
        Vf=22;
    end
end
if(sector==14)
    if(Hs==1 && Hmd==1)
        Vt=30;
        Vf=28;
     elseif(Hs==1 && Hmd==0)
        Vt=0;
        Vf=0;
    elseif(Hs==1 && Hmd==-1)
        Vt=25;
        Vf=28;
    elseif(Hs==-1 && Hmd==1)
        Vt=30;
        Vf=23;
    elseif(Hs==-1 && Hmd==0)
       Vt=31;
        Vf=31;
    else
        Vt=25;
        Vf=23;
    end
end
if(sector==15)
    if(Hs==1 && Hmd==1)
        Vt=21;
        Vf=28;
     elseif(Hs==1 && Hmd==0)
        Vt=31;
        Vf=31;
    elseif(Hs==1 && Hmd==-1)
        Vt=26;
        Vf=28;
    elseif(Hs==-1 && Hmd==1)
        Vt=21;
        Vf=23;
    elseif(Hs==-1 && Hmd==0)
       Vt=0;
        Vf=0;
    else
        Vt=26;
        Vf=23;
    end
end
if(sector==16)
    if(Hs==1 && Hmd==1)
        Vt=21;
        Vf=29;
     elseif(Hs==1 && Hmd==0)
        Vt=0;
        Vf=0;
    elseif(Hs==1 && Hmd==-1)
        Vt=26;
        Vf=29;
    elseif(Hs==-1 && Hmd==1)
        Vt=21;
        Vf=24;
    elseif(Hs==-1 && Hmd==0)
       Vt=31;
        Vf=31;
    else
        Vt=26;
        Vf=24;
    end
end
if(sector==17)
    if(Hs==1 && Hmd==1)
        Vt=22;
        Vf=29;
     elseif(Hs==1 && Hmd==0)
        Vt=31;
        Vf=31;
    elseif(Hs==1 && Hmd==-1)
        Vt=27;
        Vf=29;
    elseif(Hs==-1 && Hmd==1)
        Vt=22;
        Vf=24;
    elseif(Hs==-1 && Hmd==0)
       Vt=0;
        Vf=0;
    else
        Vt=27;
        Vf=24;
    end
end
if(sector==18)
    if(Hs==1 && Hmd==1)
        Vt=22;
        Vf=30;
     elseif(Hs==1 && Hmd==0)
        Vt=0;
        Vf=0;
    elseif(Hs==1 && Hmd==-1)
        Vt=27;
        Vf=30;
    elseif(Hs==-1 && Hmd==1)
        Vt=22;
        Vf=25;
    elseif(Hs==-1 && Hmd==0)
       Vt=31;
        Vf=31;
    else
        Vt=27;
        Vf=25;
    end
end
if(sector==19)
    if(Hs==1 && Hmd==1)
        Vt=23;
        Vf=30;
     elseif(Hs==1 && Hmd==0)
        Vt=31;
        Vf=31;
    elseif(Hs==1 && Hmd==-1)
        Vt=28;
        Vf=30;
    elseif(Hs==-1 && Hmd==1)
        Vt=23;
        Vf=25;
    elseif(Hs==-1 && Hmd==0)
       Vt=0;
        Vf=0;
    else
        Vt=28;
        Vf=25;
    end
end
if(sector==20)
    if(Hs==1 && Hmd==1)
        Vt=23;
        Vf=21;
     elseif(Hs==1 && Hmd==0)
        Vt=0;
        Vf=0;
    elseif(Hs==1 && Hmd==-1)
        Vt=28;
        Vf=21;
    elseif(Hs==-1 && Hmd==1)
        Vt=23;
        Vf=26;
    elseif(Hs==-1 && Hmd==0)
       Vt=31;
        Vf=31;
    else
        Vt=28;
        Vf=26;
    end
end
end
% Medium speed of operation
if(abs(W)>100 && abs(W)<=200)
if(sector==1)
     if(Hs==1 && Hmd==1)
        Vt=14;
        Vf=11;
     elseif(Hs==1 && Hmd==0)
        Vt=31;
        Vf=31;
    elseif(Hs==1 && Hmd==-1)
        Vt=19;
        Vf=11;
    elseif(Hs==-1 && Hmd==1)
        Vt=14;
        Vf=16;
    elseif(Hs==-1 && Hmd==0)
        Vt=0;
        Vf=0;
    else
        Vt=19;
        Vf=16;
    end
 end
if(sector==2)
    if(Hs==1 && Hmd==1)
        Vt=14;
        Vf=12;
     elseif(Hs==1 && Hmd==0)
        Vt=0;
        Vf=0;
    elseif(Hs==1 && Hmd==-1)
        Vt=19;
        Vf=12;
    elseif(Hs==-1 && Hmd==1)
        Vt=14;
        Vf=17;
    elseif(Hs==-1 && Hmd==0)
        Vt=31;
        Vf=31;
    else
        Vt=19;
        Vf=17;
    end
end
if(sector==3)
    if(Hs==1 && Hmd==1)
        Vt=15;
        Vf=12;
     elseif(Hs==1 && Hmd==0)
        Vt=31;
        Vf=31;
    elseif(Hs==1 && Hmd==-1)
        Vt=20;
        Vf=12;
    elseif(Hs==-1 && Hmd==1)
        Vt=15;
        Vf=17;
    elseif(Hs==-1 && Hmd==0)
        Vt=0;
        Vf=0;
    else
        Vt=20;
        Vf=17;
    end
end
if(sector==4)
    if(Hs==1 && Hmd==1)
        Vt=15;
        Vf=13;
     elseif(Hs==1 && Hmd==0)
        Vt=0;
        Vf=0;
    elseif(Hs==1 && Hmd==-1)
        Vt=20;
        Vf=13;
    elseif(Hs==-1 && Hmd==1)
        Vt=15;
        Vf=18;
    elseif(Hs==-1 && Hmd==0)
        Vt=31;
        Vf=31;
    else
        Vt=20;
        Vf=18;
    end
end
if(sector==5)
    if(Hs==1 && Hmd==1)
        Vt=16;
        Vf=13;
     elseif(Hs==1 && Hmd==0)
        Vt=31;
        Vf=31;
    elseif(Hs==1 && Hmd==-1)
        Vt=11;
        Vf=13;
    elseif(Hs==-1 && Hmd==1)
        Vt=16;
        Vf=18;
    elseif(Hs==-1 && Hmd==0)
        Vt=0;
        Vf=0;
    else
        Vt=11;
        Vf=18;
    end
end
if(sector==6)
    if(Hs==1 && Hmd==1)
        Vt=16;
        Vf=14;
     elseif(Hs==1 && Hmd==0)
        Vt=0;
        Vf=0;
    elseif(Hs==1 && Hmd==-1)
        Vt=11;
        Vf=14;
    elseif(Hs==-1 && Hmd==1)
        Vt=16;
        Vf=19;
    elseif(Hs==-1 && Hmd==0)
        Vt=31;
        Vf=31;
    else
        Vt=11;
        Vf=19;
    end
end
if(sector==7)
    if(Hs==1 && Hmd==1)
        Vt=17;
        Vf=14;
     elseif(Hs==1 && Hmd==0)
        Vt=31;
        Vf=31;
    elseif(Hs==1 && Hmd==-1)
        Vt=12;
        Vf=14;
    elseif(Hs==-1 && Hmd==1)
        Vt=17;
        Vf=19;
    elseif(Hs==-1 && Hmd==0)
        Vt=0;
        Vf=0;
    else
        Vt=12;
        Vf=19;
    end
end
if(sector==8)
    if(Hs==1 && Hmd==1)
        Vt=17;
        Vf=15;
     elseif(Hs==1 && Hmd==0)
        Vt=0;
        Vf=0;
    elseif(Hs==1 && Hmd==-1)
        Vt=12;
        Vf=15;
    elseif(Hs==-1 && Hmd==1)
        Vt=17;
        Vf=20;
    elseif(Hs==-1 && Hmd==0)
        Vt=31;
        Vf=31;
    else
        Vt=12;
        Vf=20;
    end
end
if(sector==9)
    if(Hs==1 && Hmd==1)
        Vt=18;
        Vf=15;
     elseif(Hs==1 && Hmd==0)
        Vt=31;
        Vf=31;
    elseif(Hs==1 && Hmd==-1)
        Vt=13;
        Vf=15;
    elseif(Hs==-1 && Hmd==1)
        Vt=18;
        Vf=20;
    elseif(Hs==-1 && Hmd==0)
        Vt=0;
        Vf=0;
    else
        Vt=13;
        Vf=20;
    end
end
if(sector==10)
    if(Hs==1 && Hmd==1)
        Vt=18;
        Vf=16;
     elseif(Hs==1 && Hmd==0)
        Vt=0;
        Vf=0;
    elseif(Hs==1 && Hmd==-1)
        Vt=13;
        Vf=16;
    elseif(Hs==-1 && Hmd==1)
        Vt=18;
        Vf=11;
    elseif(Hs==-1 && Hmd==0)
       Vt=31;
        Vf=31;
    else
        Vt=13;
        Vf=11;
    end
end
if(sector==11)
    if(Hs==1 && Hmd==1)
        Vt=19;
        Vf=16;
     elseif(Hs==1 && Hmd==0)
        Vt=31;
        Vf=31;
    elseif(Hs==1 && Hmd==-1)
        Vt=14;
        Vf=16;
    elseif(Hs==-1 && Hmd==1)
        Vt=19;
        Vf=11;
    elseif(Hs==-1 && Hmd==0)
       Vt=0;
        Vf=0;
    else
        Vt=14;
        Vf=11;
    end
end
if(sector==12)
    if(Hs==1 && Hmd==1)
        Vt=19;
        Vf=17;
     elseif(Hs==1 && Hmd==0)
        Vt=0;
        Vf=0;
    elseif(Hs==1 && Hmd==-1)
        Vt=14;
        Vf=17;
    elseif(Hs==-1 && Hmd==1)
        Vt=19;
        Vf=12;
    elseif(Hs==-1 && Hmd==0)
       Vt=31;
        Vf=31;
    else
        Vt=14;
        Vf=12;
    end
end
if(sector==13)
    if(Hs==1 && Hmd==1)
        Vt=20;
        Vf=17;
     elseif(Hs==1 && Hmd==0)
        Vt=31;
        Vf=31;
    elseif(Hs==1 && Hmd==-1)
        Vt=15;
        Vf=17;
    elseif(Hs==-1 && Hmd==1)
        Vt=20;
        Vf=12;
    elseif(Hs==-1 && Hmd==0)
       Vt=0;
        Vf=0;
    else
        Vt=15;
        Vf=12;
    end
end
if(sector==14)
    if(Hs==1 && Hmd==1)
        Vt=20;
        Vf=18;
     elseif(Hs==1 && Hmd==0)
        Vt=0;
        Vf=0;
    elseif(Hs==1 && Hmd==-1)
        Vt=15;
        Vf=18;
    elseif(Hs==-1 && Hmd==1)
        Vt=20;
        Vf=13;
    elseif(Hs==-1 && Hmd==0)
       Vt=31;
        Vf=31;
    else
        Vt=15;
        Vf=13;
    end
end
if(sector==15)
    if(Hs==1 && Hmd==1)
        Vt=11;
        Vf=18;
     elseif(Hs==1 && Hmd==0)
        Vt=31;
        Vf=31;
    elseif(Hs==1 && Hmd==-1)
        Vt=16;
        Vf=18;
    elseif(Hs==-1 && Hmd==1)
        Vt=11;
        Vf=13;
    elseif(Hs==-1 && Hmd==0)
       Vt=0;
        Vf=0;
    else
        Vt=16;
        Vf=13;
    end
end
if(sector==16)
    if(Hs==1 && Hmd==1)
        Vt=11;
        Vf=19;
     elseif(Hs==1 && Hmd==0)
        Vt=0;
        Vf=0;
    elseif(Hs==1 && Hmd==-1)
        Vt=16;
        Vf=19;
    elseif(Hs==-1 && Hmd==1)
        Vt=11;
        Vf=14;
    elseif(Hs==-1 && Hmd==0)
       Vt=31;
        Vf=31;
    else
        Vt=16;
        Vf=14;
    end
end
if(sector==17)
    if(Hs==1 && Hmd==1)
        Vt=12;
        Vf=19;
     elseif(Hs==1 && Hmd==0)
        Vt=31;
        Vf=31;
    elseif(Hs==1 && Hmd==-1)
        Vt=17;
        Vf=19;
    elseif(Hs==-1 && Hmd==1)
        Vt=12;
        Vf=14;
    elseif(Hs==-1 && Hmd==0)
       Vt=0;
        Vf=0;
    else
        Vt=17;
        Vf=14;
    end
end
if(sector==18)
    if(Hs==1 && Hmd==1)
        Vt=12;
        Vf=20;
     elseif(Hs==1 && Hmd==0)
        Vt=0;
        Vf=0;
    elseif(Hs==1 && Hmd==-1)
        Vt=17;
        Vf=20;
    elseif(Hs==-1 && Hmd==1)
        Vt=12;
        Vf=15;
    elseif(Hs==-1 && Hmd==0)
       Vt=31;
        Vf=31;
    else
        Vt=17;
        Vf=15;
    end
end
if(sector==19)
    if(Hs==1 && Hmd==1)
        Vt=13;
        Vf=20;
     elseif(Hs==1 && Hmd==0)
        Vt=31;
        Vf=31;
    elseif(Hs==1 && Hmd==-1)
        Vt=18;
        Vf=20;
    elseif(Hs==-1 && Hmd==1)
        Vt=13;
        Vf=15;
    elseif(Hs==-1 && Hmd==0)
       Vt=0;
        Vf=0;
    else
        Vt=18;
        Vf=15;
    end
end
if(sector==20)
    if(Hs==1 && Hmd==1)
        Vt=13;
        Vf=11;
     elseif(Hs==1 && Hmd==0)
        Vt=0;
        Vf=0;
    elseif(Hs==1 && Hmd==-1)
        Vt=18;
        Vf=11;
    elseif(Hs==-1 && Hmd==1)
        Vt=13;
        Vf=16;
    elseif(Hs==-1 && Hmd==0)
       Vt=31;
        Vf=31;
    else
        Vt=18;
        Vf=16;
    end
end
end
% High speed of operation
if(abs(W)>200 && abs(W)<=314)
 if(sector==1)
     if(Hs==1 && Hmd==1)
        Vt=4;
        Vf=1;
     elseif(Hs==1 && Hmd==0)
        Vt=31;
        Vf=31;
    elseif(Hs==1 && Hmd==-1)
        Vt=9;
        Vf=1;
    elseif(Hs==-1 && Hmd==1)
        Vt=4;
        Vf=6;
    elseif(Hs==-1 && Hmd==0)
        Vt=0;
        Vf=0;
    else
        Vt=9;
        Vf=6;
    end
 end
if(sector==2)
    if(Hs==1 && Hmd==1)
        Vt=4;
        Vf=2;
     elseif(Hs==1 && Hmd==0)
        Vt=0;
        Vf=0;
    elseif(Hs==1 && Hmd==-1)
        Vt=9;
        Vf=2;
    elseif(Hs==-1 && Hmd==1)
        Vt=4;
        Vf=7;
    elseif(Hs==-1 && Hmd==0)
        Vt=31;
        Vf=31;
    else
        Vt=9;
        Vf=7;
    end
end
if(sector==3)
    if(Hs==1 && Hmd==1)
        Vt=5;
        Vf=2;
     elseif(Hs==1 && Hmd==0)
        Vt=31;
        Vf=31;
    elseif(Hs==1 && Hmd==-1)
        Vt=10;
        Vf=2;
    elseif(Hs==-1 && Hmd==1)
        Vt=5;
        Vf=7;
    elseif(Hs==-1 && Hmd==0)
        Vt=0;
        Vf=0;
    else
        Vt=10;
        Vf=7;
    end
end
if(sector==4)
    if(Hs==1 && Hmd==1)
        Vt=5;
        Vf=3;
     elseif(Hs==1 && Hmd==0)
        Vt=0;
        Vf=0;
    elseif(Hs==1 && Hmd==-1)
        Vt=10;
        Vf=3;
    elseif(Hs==-1 && Hmd==1)
        Vt=5;
        Vf=8;
    elseif(Hs==-1 && Hmd==0)
        Vt=31;
        Vf=31;
    else
        Vt=10;
        Vf=8;
    end
end
if(sector==5)
    if(Hs==1 && Hmd==1)
        Vt=6;
        Vf=3;
     elseif(Hs==1 && Hmd==0)
        Vt=31;
        Vf=31;
    elseif(Hs==1 && Hmd==-1)
        Vt=1;
        Vf=3;
    elseif(Hs==-1 && Hmd==1)
        Vt=6;
        Vf=8;
    elseif(Hs==-1 && Hmd==0)
        Vt=0;
        Vf=0;
    else
        Vt=1;
        Vf=8;
    end
end
if(sector==6)
    if(Hs==1 && Hmd==1)
        Vt=6;
        Vf=4;
     elseif(Hs==1 && Hmd==0)
        Vt=0;
        Vf=0;
    elseif(Hs==1 && Hmd==-1)
        Vt=1;
        Vf=4;
    elseif(Hs==-1 && Hmd==1)
        Vt=6;
        Vf=9;
    elseif(Hs==-1 && Hmd==0)
        Vt=31;
        Vf=31;
    else
        Vt=1;
        Vf=9;
    end
end
if(sector==7)
    if(Hs==1 && Hmd==1)
        Vt=7;
        Vf=4;
     elseif(Hs==1 && Hmd==0)
        Vt=31;
        Vf=31;
    elseif(Hs==1 && Hmd==-1)
        Vt=2;
        Vf=4;
    elseif(Hs==-1 && Hmd==1)
        Vt=7;
        Vf=9;
    elseif(Hs==-1 && Hmd==0)
        Vt=0;
        Vf=0;
    else
        Vt=2;
        Vf=9;
    end
end
if(sector==8)
    if(Hs==1 && Hmd==1)
        Vt=7;
        Vf=5;
     elseif(Hs==1 && Hmd==0)
        Vt=0;
        Vf=0;
    elseif(Hs==1 && Hmd==-1)
        Vt=2;
        Vf=5;
    elseif(Hs==-1 && Hmd==1)
        Vt=7;
        Vf=10;
    elseif(Hs==-1 && Hmd==0)
        Vt=31;
        Vf=31;
    else
        Vt=2;
        Vf=10;
    end
end
if(sector==9)
    if(Hs==1 && Hmd==1)
        Vt=8;
        Vf=5;
     elseif(Hs==1 && Hmd==0)
        Vt=31;
        Vf=31;
    elseif(Hs==1 && Hmd==-1)
        Vt=3;
        Vf=5;
    elseif(Hs==-1 && Hmd==1)
        Vt=8;
        Vf=10;
    elseif(Hs==-1 && Hmd==0)
        Vt=0;
        Vf=0;
    else
        Vt=3;
        Vf=10;
    end
end
if(sector==10)
    if(Hs==1 && Hmd==1)
        Vt=8;
        Vf=6;
     elseif(Hs==1 && Hmd==0)
        Vt=0;
        Vf=0;
    elseif(Hs==1 && Hmd==-1)
        Vt=3;
        Vf=6;
    elseif(Hs==-1 && Hmd==1)
        Vt=8;
        Vf=1;
    elseif(Hs==-1 && Hmd==0)
       Vt=31;
        Vf=31;
    else
        Vt=3;
        Vf=1;
    end
end
if(sector==11)
    if(Hs==1 && Hmd==1)
        Vt=9;
        Vf=6;
     elseif(Hs==1 && Hmd==0)
        Vt=31;
        Vf=31;
    elseif(Hs==1 && Hmd==-1)
        Vt=4;
        Vf=6;
    elseif(Hs==-1 && Hmd==1)
        Vt=9;
        Vf=1;
    elseif(Hs==-1 && Hmd==0)
       Vt=0;
        Vf=0;
    else
        Vt=4;
        Vf=1;
    end
end
if(sector==12)
    if(Hs==1 && Hmd==1)
        Vt=9;
        Vf=7;
     elseif(Hs==1 && Hmd==0)
        Vt=0;
        Vf=0;
    elseif(Hs==1 && Hmd==-1)
        Vt=4;
        Vf=7;
    elseif(Hs==-1 && Hmd==1)
        Vt=9;
        Vf=2;
    elseif(Hs==-1 && Hmd==0)
       Vt=31;
        Vf=31;
    else
        Vt=4;
        Vf=2;
    end
end
if(sector==13)
    if(Hs==1 && Hmd==1)
        Vt=10;
        Vf=7;
     elseif(Hs==1 && Hmd==0)
        Vt=31;
        Vf=31;
    elseif(Hs==1 && Hmd==-1)
        Vt=5;
        Vf=7;
    elseif(Hs==-1 && Hmd==1)
        Vt=10;
        Vf=2;
    elseif(Hs==-1 && Hmd==0)
       Vt=0;
        Vf=0;
    else
        Vt=5;
        Vf=2;
    end
end
if(sector==14)
    if(Hs==1 && Hmd==1)
        Vt=10;
        Vf=8;
     elseif(Hs==1 && Hmd==0)
        Vt=0;
        Vf=0;
    elseif(Hs==1 && Hmd==-1)
        Vt=5;
        Vf=8;
    elseif(Hs==-1 && Hmd==1)
        Vt=10;
        Vf=3;
    elseif(Hs==-1 && Hmd==0)
       Vt=31;
        Vf=31;
    else
        Vt=5;
        Vf=3;
    end
end
if(sector==15)
    if(Hs==1 && Hmd==1)
        Vt=1;
        Vf=8;
     elseif(Hs==1 && Hmd==0)
        Vt=31;
        Vf=31;
    elseif(Hs==1 && Hmd==-1)
        Vt=6;
        Vf=8;
    elseif(Hs==-1 && Hmd==1)
        Vt=1;
        Vf=3;
    elseif(Hs==-1 && Hmd==0)
       Vt=0;
        Vf=0;
    else
        Vt=6;
        Vf=3;
    end
end
if(sector==16)
    if(Hs==1 && Hmd==1)
        Vt=1;
        Vf=9;
     elseif(Hs==1 && Hmd==0)
        Vt=0;
        Vf=0;
    elseif(Hs==1 && Hmd==-1)
        Vt=6;
        Vf=9;
    elseif(Hs==-1 && Hmd==1)
        Vt=1;
        Vf=4;
    elseif(Hs==-1 && Hmd==0)
       Vt=31;
        Vf=31;
    else
        Vt=6;
        Vf=4;
    end
end
if(sector==17)
    if(Hs==1 && Hmd==1)
        Vt=2;
        Vf=9;
     elseif(Hs==1 && Hmd==0)
        Vt=31;
        Vf=31;
    elseif(Hs==1 && Hmd==-1)
        Vt=7;
        Vf=9;
    elseif(Hs==-1 && Hmd==1)
        Vt=2;
        Vf=4;
    elseif(Hs==-1 && Hmd==0)
       Vt=0;
        Vf=0;
    else
        Vt=7;
        Vf=4;
    end
end
if(sector==18)
    if(Hs==1 && Hmd==1)
        Vt=2;
        Vf=10;
     elseif(Hs==1 && Hmd==0)
        Vt=0;
        Vf=0;
    elseif(Hs==1 && Hmd==-1)
        Vt=7;
        Vf=10;
    elseif(Hs==-1 && Hmd==1)
        Vt=2;
        Vf=5;
    elseif(Hs==-1 && Hmd==0)
       Vt=31;
        Vf=31;
    else
        Vt=7;
        Vf=5;
    end
end
if(sector==19)
    if(Hs==1 && Hmd==1)
        Vt=3;
        Vf=10;
     elseif(Hs==1 && Hmd==0)
        Vt=31;
        Vf=31;
    elseif(Hs==1 && Hmd==-1)
        Vt=8;
        Vf=10;
    elseif(Hs==-1 && Hmd==1)
        Vt=3;
        Vf=5;
    elseif(Hs==-1 && Hmd==0)
       Vt=0;
        Vf=0;
    else
        Vt=8;
        Vf=5;
    end
end
if(sector==20)
    if(Hs==1 && Hmd==1)
        Vt=3;
        Vf=1;
     elseif(Hs==1 && Hmd==0)
        Vt=0;
        Vf=0;
    elseif(Hs==1 && Hmd==-1)
        Vt=8;
        Vf=1;
    elseif(Hs==-1 && Hmd==1)
        Vt=3;
        Vf=6;
    elseif(Hs==-1 && Hmd==0)
       Vt=31;
        Vf=31;
    else
        Vt=8;
        Vf=6;
    end
end
end

== matlab function FP_PMSM_ProposedDTC/Controller/MATLAB Function5 ==
  data: G input; v output; S input
function v  = fcn(G,S)
v=0;
if (G==1)
  if (S==9) || (S==10) ||(S==1)  || (S==2) ||(S==3)
     v=1;
  elseif(S==4) || (S==5) ||(S==6)  || (S==7) ||(S==8)
     v=11;
  end
elseif (G==2)
  if (S==2) || (S==3) ||(S==4)  || (S==5) ||(S==6)
     v=2;
  elseif(S==7) || (S==8) ||(S==9)  || (S==10) ||(S==1)
     v=12;
  end
elseif (G==3)
  if (S==5) || (S==6) ||(S==7)  || (S==8) ||(S==9)
     v=3;
  elseif(S==10) || (S==1) ||(S==2)  || (S==3) ||(S==4)
     v=13;
  end
elseif (G==4)
  if (S==8) || (S==9) ||(S==10)  || (S==1) ||(S==2)
     v=4;
  elseif(S==3) || (S==4) ||(S==5)  || (S==6) ||(S==7)
     v=14;
  end
elseif (G==5)
  if (S==1) || (S==2) ||(S==3)  || (S==4) ||(S==5)
     v=5;
  elseif(S==6) || (S==7) ||(S==8)  || (S==9) ||(S==10)
     v=15;
  end  
elseif (G==6)
  if (S==4) || (S==5) ||(S==6)  || (S==7) ||(S==8)
     v=6;
  elseif(S==9) || (S==10) ||(S==1)  || (S==2) ||(S==3)
     v=16;
  end
elseif (G==7)
  if (S==7) || (S==8) ||(S==9)  || (S==10) ||(S==1)
     v=7;
  elseif(S==2) || (S==3) ||(S==4)  || (S==5) ||(S==6)
     v=17;
  end
elseif (G==8)
  if (S==10) || (S==1) ||(S==2)  || (S==3) ||(S==4)
     v=8;
  elseif (S==5) ||(S==6)  || (S==7) ||(S==8)|| (S==9)
     v=18;
  end
elseif (G==9)
  if (S==3) || (S==4) ||(S==5)  || (S==6) ||(S==7)
     v=9;
  elseif(S==8) || (S==9) ||(S==10)  || (S==1) ||(S==2)
     v=19;
  end  
 elseif (G==10)
  if (S==6) || (S==7) ||(S==8)  || (S==9) ||(S==10)
     v=10;
  elseif(S==1) || (S==2) || (S==3) ||(S==4)  || (S==5)
     v=20;
  end
end

== matlab function FP_PMSM_ProposedDTC/Frequency measurement/MATLAB Function1 ==
  data: c input; f output; p input
function f  = fcn(c,p)
persistent k s 
if isempty(k), k = 1; end
if isempty(s), s = 0; end
if (c>=1 && c<=2)
    if (k~=p)
        k=p;
        s=s+1;
    end
end
f = s/2;

== matlab function FP_PMSM_ProposedDTC/Frequency measurement/MATLAB Function2 ==
  data: c input; f output; p input
function f  = fcn(c,p)
persistent k s 
if isempty(k), k = 1; end
if isempty(s), s = 0; end
if (c>=1 && c<=2)
    if (k~=p)
        k=p;
        s=s+1;
    end
end
f = s/2;

== matlab function FP_PMSM_ProposedDTC/Frequency measurement/MATLAB Function3 ==
  data: c input; f output; p input
function f  = fcn(c,p)
persistent k s 
if isempty(k), k = 1; end
if isempty(s), s = 0; end
if (c>=1 && c<=2)
    if (k~=p)
        k=p;
        s=s+1;
    end
end
f = s/2;

== matlab function FP_PMSM_ProposedDTC/Frequency measurement/MATLAB Function4 ==
  data: c input; f output; p input
function f  = fcn(c,p)
persistent k s 
if isempty(k), k = 1; end
if isempty(s), s = 0; end
if (c>=1 && c<=2)
    if (k~=p)
        k=p;
        s=s+1;
    end
end
f = s/2;

== matlab function FP_PMSM_ProposedDTC/Frequency measurement/MATLAB Function5 ==
  data: c input; f output; p input
function f  = fcn(c,p)
persistent k s 
if isempty(k), k = 1; end
if isempty(s), s = 0; end
if (c>=1 && c<=2)
    if (k~=p)
        k=p;
        s=s+1;
    end
end
f = s/2;

== matlab function FP_PMSM_ProposedDTC/Controller/Duty Calculation ==
  data: Vt input; Df output; Dt output; Vf input; thetaT input; thetaF input; theta1 input; theta2 input; Fsref input; Fsactual input; Tref input; Iss input
function [Df,Dt] = fcn(Vt,Vf,thetaT,thetaF,theta1,theta2,Fsref,Fsactual,Tref,Iss)
P=4;
Ls=0.022;
Lamda_PM=0.5;
Ts=40e-6;
A=(Vt)*Ts*cos(thetaT-theta1);
B=(Vf)*Ts*cos(thetaF-theta1);
M=(Vt)*Ts*sin(thetaT-theta1);
N=(Vf)*Ts*sin(thetaF-theta1);
K=Fsref-Fsactual;
Q=Ls*((Tref*4)/(5*P*Lamda_PM)-Iss*sin(theta2-theta1));
Df=abs((M*K-A*Q)/(B*M-N*A));
Dt=abs((B*Q-N*K)/(B*M-N*A));
if(Df>=1)
    Df=1;
end
if(Dt>=1)
    Dt=1;
end
